simulink model "Task3_Structured_Residuals"  (R2023a)
settings: Solver=ode5  StartTime=0.0  StopTime=15  FixedStep=0.025  RelTol=1e-3  EnableMultiTasking=on
libraries: simulink x3
settings Model: Creator=Guptas  LastModifiedBy=Guptas
settings DataIOCC: LimitDataPoints=on  SaveFormat=Array  SignalLoggingSaveFormat=ModelDataLogs  ReturnWorkspaceOutputs=off  SignalLoggingName=sigsOut
settings OptimizationCC: BlockReduction=off  BooleanDataType=off
settings DebuggingCC: SaveWithParameterizedLinksMsg=none  UnderspecifiedInitializationDetection=Classic  MergeDetectMultiDrivingBlocksExec=none  SignalResolutionControl=TryResolveAllWithWarning  MultiTaskDSMMsg=warning  MultiTaskCondExecSysMsg=none  UnconnectedInputMsg=warning  UnconnectedOutputMsg=warning  UnconnectedLineMsg=warning
settings HardwareCC: ProdBitPerPointer=32  ProdBitPerSizeT=32  ProdBitPerPtrDiffT=32  ProdLargestAtomicFloat=None  ProdIntDivRoundTo=Undefined  ProdEndianess=Unspecified  ProdWordSize=32  ProdHWDeviceType=32-bit Generic  TargetUnknown=on
settings ModelReferenceCC: PropagateSignalLabelsOutOfModel=off
settings GRTTargetCC: CombineOutputUpdateFcns=off  GRTInterface=on
settings ConfigComp: CovMetricSettings=dw  CovSaveCumulativeToWorkspaceVar=on  CovSaveSingleToWorkspaceVar=on

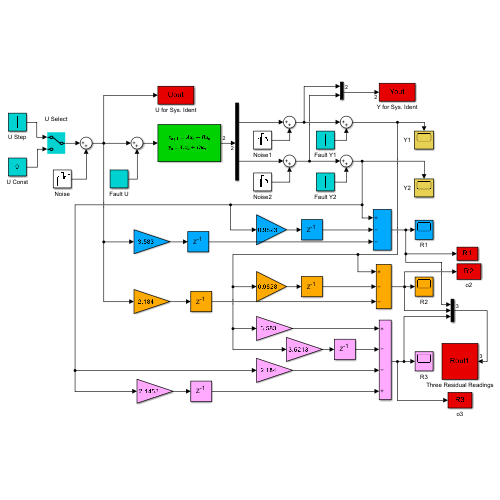
[thumbnail: Simulink's stored preview of the top-level diagram]
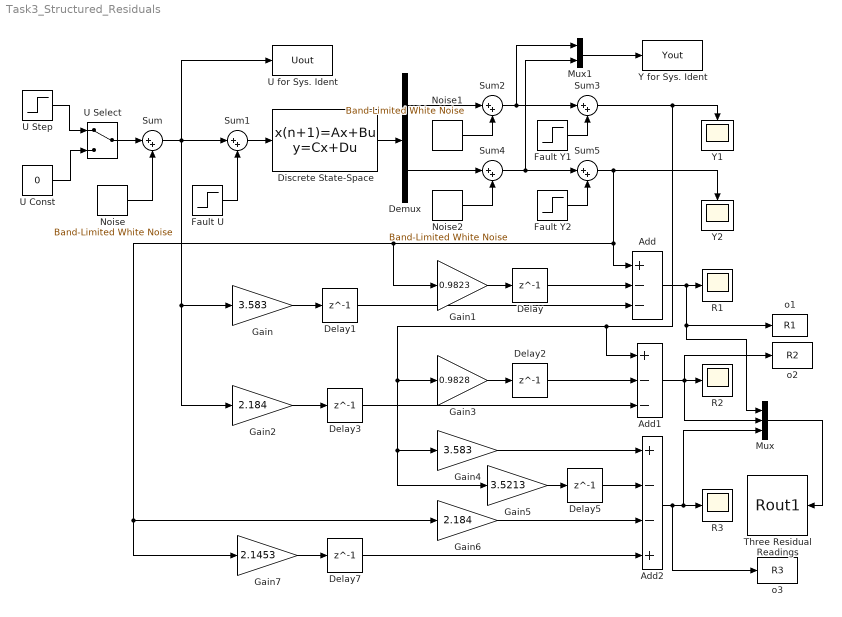
== system Task3_Structured_Residuals ==
  Add : Sum  Inputs=+--
  Add1 : Sum  Inputs=+--
  Add2 : Sum  Inputs=+--+
  Delay{,1..3,5,7} (6 alike) : Delay  DelayLength=1  InitialCondition=0
  Demux : Demux  Outputs=2
      settings: DisplayOption=none
  Discrete State-Space : DiscreteStateSpace  A=|  B=|  C=[1 0; 0 1]  D=[0;0]  SampleTime=0.025
      A=|
      | [0.9769 0.0038;
      | 0.0936 0.9225]
      B=|
      | [2.1521;
      | 3.8186]
  Fault U : Step  Time=3  After=0  SampleTime=0
  Fault Y1 : Step  Time=3  After=5  SampleTime=0
  Fault Y2 : Step  Time=3  After=5  SampleTime=0
  Gain : Gain  Gain=3.583
  Gain1 : Gain  Gain=0.9823
  Gain2 : Gain  Gain=2.184
  Gain3 : Gain  Gain=0.9828
  Gain4 : Gain  Gain=3.583
  Gain5 : Gain  Gain=3.5213
  Gain6 : Gain  Gain=2.184
  Gain7 : Gain  Gain=2.1453
  Mux : Mux  Inputs=3
  Mux1 : Mux  Inputs=2
  Noise : simulink/Sources/Band-Limited White Noise  Cov=[0.01]  Ts=0.025  seed=[23341]
  Noise1 : simulink/Sources/Band-Limited White Noise  Cov=[0.1]  Ts=0.025  seed=[23341]
  Noise2 : simulink/Sources/Band-Limited White Noise  Cov=[0.1]  Ts=0.025  seed=[23341]
  R1 : Scope
  R2 : Scope
  R3 : Scope
  Sum{,1..5} (6 alike) : Sum  Inputs=|++  SaturateOnIntegerOverflow=on
  Three Residual Readings : ToWorkspace  VariableName=Rout1  SampleTime=0.025
  U Const : Constant  Value=0
  "U Select " : ManualSwitch
  U Step : Step  SampleTime=0
  U for Sys. Ident : ToWorkspace  VariableName=Uout  SampleTime=0.025
  Y for Sys. Ident : ToWorkspace  VariableName=Yout  SampleTime=0.025
  Y1 : Scope
  Y2 : Scope
  o1 : ToWorkspace  VariableName=R1  SampleTime=0.025
  o2 : ToWorkspace  VariableName=R2  SampleTime=0.025
  o3 : ToWorkspace  VariableName=R3  SampleTime=0.025
  wires:
  U Const/1 -> "U Select "/2
  U Step/1 -> "U Select "/1
  Mux1/1 -> Y for Sys. Ident/1
  Discrete State-Space/1 -> Demux/1
  Sum/1 -> Gain2/1, Gain/1, Sum1/1, U for Sys. Ident/1
  Sum1/1 -> Discrete State-Space/1
  "U Select "/1 -> Sum/1
  Sum2/1 -> Sum3/1, Mux1/1
  Sum4/1 -> Sum5/1, Mux1/2
  Sum3/1 -> Add1/1, Gain3/1, Gain5/1, Gain4/1, Y1/1
  Sum5/1 -> Y2/1, Gain7/1, Gain6/1, Gain1/1, Add/1
  Demux/1 -> Sum2/1
  Demux/2 -> Sum4/1
  Gain1/1 -> Delay/1
  Gain/1 -> Delay1/1
  Add/1 -> Mux/1, o1/1, R1/1
  Delay/1 -> Add/2
  Delay1/1 -> Add/3
  Add1/1 -> Mux/2, o2/1, R2/1
  Gain2/1 -> Delay3/1
  Gain3/1 -> Delay2/1
  Delay2/1 -> Add1/2
  Delay3/1 -> Add1/3
  Add2/1 -> o3/1, Mux/3, R3/1
  Gain5/1 -> Delay5/1
  Gain7/1 -> Delay7/1
  Delay7/1 -> Add2/4
  Gain4/1 -> Add2/1
  Delay5/1 -> Add2/2
  Mux/1 -> Three Residual Readings/1
  Gain6/1 -> Add2/3
  Noise/1 -> Sum/2
  Noise1/1 -> Sum2/2
  Noise2/1 -> Sum4/2
  Fault U/1 -> Sum1/2
  Fault Y1/1 -> Sum3/2
  Fault Y2/1 -> Sum5/2
